simulink model "psbloadshed"  (Simulink 6.0)
settings: Solver=ode23tb  SolverMode=SingleTasking  StartTime=0.0  StopTime=2  RelTol=1e-3
InitFcn:
  | powericon('psbinitsys',bdroot);
libraries: powerlib2 x9, simulink x1
settings Model: Creator=patrice  LastModifiedBy=batserve  ExtModeTrigMode=oneshot  ExtModeArmWhenConnect=off  ExtModeAutoUpdateStatusClock=off
settings DataIOCC: LimitDataPoints=off  SignalLoggingName=sigsOut
settings OptimizationCC: BlockReduction=off  BooleanDataType=off
settings DebuggingCC: CheckExecutionContextPreStartOutputMsg=on  CheckExecutionContextRuntimeOutputMsg=on  SolverPrmCheckMsg=none  IntegerOverflowMsg=none
settings HardwareCC: TargetUnknown=on
settings RTWCC: TemplateMakefile=grt_unix.tmf

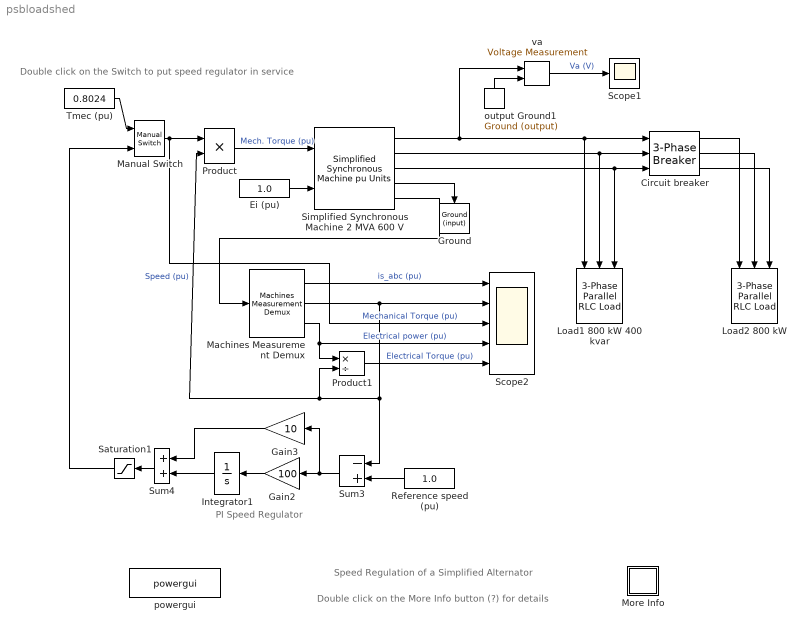
== system psbloadshed ==
  note: Speed Regulation of a Simplified Alternator
  note: Double click on the More Info button (?) for details
  note: PI Speed Regulator
  note: Double click on the  Switch
      | to put speed regulator
      | in service
  Circuit breaker : powerlib2/Elements/3-Phase Breaker  init_states=closed  sa=on  sb=on  sc=on  sw_times=[ 0.2 0.7*100 ]  Ts=0  comext=off  Ron=1e-4  Rp=inf  Cp=0  mesure=None
  Ei (pu) : Constant  Value=1.0
  Gain2 : Gain  Orientation=left  Gain=100  SaturateOnIntegerOverflow=on
  Gain3 : Gain  Orientation=left  Gain=10  SaturateOnIntegerOverflow=on
  Ground : powerlib2/Connectors/Ground (input)  Tag=PoWeRsYsTeMbLoCk  Orientation=down
  Integrator1 : Integrator  Orientation=left  InitialCondition=0.8024  LimitOutput=on  UpperSaturationLimit=1  LowerSaturationLimit=0  ZeroCross=off
  Load1 800 kW 400 kvar : powerlib2/Elements/3-Phase Parallel RLC Load  Orientation=down  Vpp=600  fn=60  P3=800e3  QL3=400e3  QC3=0
  Load2 800 kW : powerlib2/Elements/3-Phase Parallel RLC Load  Orientation=down  Vpp=600  fn=60  P3=800e3  QL3=0  QC3=0
  Machines Measurement Demux : powerlib2/Machines/Machines Measurement Demux  machType=Simplified synchronous  ssm1=on  ssm2=off  ssm3=off  ssm4=off  ssm5=on  ssm6=on  sm1=on  sm2=on  sm3=on  sm4=on  sm5=on  sm6=on  sm7=on  sm8=on  sm9=on  sm10=on  sm11=on  sm115=off  sm12=off  sm13=off  sm14=off  asm1=on  asm2=on  asm3=on  asm4=on  asm5=on  asm6=on  asm7=on  asm8=on  asm9=on  asm10=on  asm11=on  pmsm1=on  pmsm2=on  pmsm3=on  pmsm4=on  pmsm5=on  pmsm6=on  lastType=1
  Manual Switch : simulink/Signal Routing/Manual Switch  sw=1  action=0
  More Info : Subsystem
      mask Display: disp('?')
  Product : Product  SaturateOnIntegerOverflow=on  InputSameDT=on
  Product1 : Product  Inputs=*/  SaturateOnIntegerOverflow=on  InputSameDT=on
  Reference speed (pu) : Constant  Orientation=left  Value=1.0
  Saturation1 : Saturate  Orientation=left  UpperLimit=1  LowerLimit=0  ZeroCross=off
  "Scope1 " : Scope
      settings: TimeRange=0.2  YMin=-500  YMax=500  DataFormat=Structure
  Scope2 : Scope  NumInputPorts=5
      settings: TimeRange=2  YMin=-1~1~-2~0~0  YMax=1~2~2~1~1  DataFormat=Structure  SampleTime=1/60
  Simplified Synchronous Machine 2 MVA 600 V : powerlib2/Machines/Simplified Synchronous  Machine  pu Units  Tag=PoWeRsYsTeMbLoCk  conType=4-wire Y  x1="[  2000e3, 600, 60 ]"  x2=[ 0.6 , 0.0, 2 ]  x3="[ 0.0036  0.16 ]"  x4="[0 0  0 0 0    0  0  0]"  PSBOutputType=11110  iounits=0  LoadFlowParameters=[2 0 0 0]
  Sum3 : Sum  Orientation=left  Inputs=-+  SaturateOnIntegerOverflow=on  InputSameDT=on
  Sum4 : Sum  Orientation=left  SaturateOnIntegerOverflow=on  InputSameDT=on
  Tmec (pu) : Constant  Value=0.8024
  output Ground1 : powerlib2/Connectors/Ground (output)  Tag=PoWeRsYsTeMbLoCk  Orientation=up  PSBOutputType=1
  powergui : powerlib2/powergui  Frange=[0:2:500]  Ylog=off  Xlog=on  save=off  variable=ZData  ZoomFFT=on  StartTime=0.0  cycles=1  DisplayStyle=off  fundamental=60  FreqAxis=off  MaxFrequency=1000  frequencyindice=1  frequencyindicesteady=1  RmsSteady=1  display=off  Ts=0  methode=off  frequency=60  echomessages=off
  va : powerlib2/Measurements/Voltage Measurement  Tag=PoWeRsYsTeMmEaSuReMeNt  PhasorSimulation=off  OutputType=Magnitude  PSBOutputType=0  PSBequivalent=0
  wires:
  Simplified Synchronous Machine 2 MVA 600 V/5 -> Machines Measurement Demux/1
  Circuit breaker/1 -> Load2 800 kW/1
  Ei (pu)/1 -> Simplified Synchronous Machine 2 MVA 600 V/2
  Circuit breaker/2 -> Load2 800 kW/2
  Circuit breaker/3 -> Load2 800 kW/3
  Simplified Synchronous Machine 2 MVA 600 V/2 -> Circuit breaker/2, Load1 800 kW 400 kvar/2
  Simplified Synchronous Machine 2 MVA 600 V/3 -> Load1 800 kW 400 kvar/3, Circuit breaker/3
  Simplified Synchronous Machine 2 MVA 600 V/1 -> Circuit breaker/1, Load1 800 kW 400 kvar/1, va/1
  output Ground1/1 -> va/2
  Machines Measurement Demux/1 -> Scope2/1  "is_abc (pu)"
  Machines Measurement Demux/2 -> Scope2/2, Sum3/1, Product/2, Product1/2  "Speed (pu)"
  Gain3/1 -> Sum4/1
  Gain2/1 -> Integrator1/1
  Sum3/1 -> Gain3/1, Gain2/1
  Integrator1/1 -> Sum4/2
  Reference speed (pu)/1 -> Sum3/2
  Sum4/1 -> Saturation1/1
  Product/1 -> Simplified Synchronous Machine 2 MVA 600 V/1  "Mech. Torque (pu)"
  va/1 -> "Scope1 "/1  "Va (V)"
  Tmec (pu)/1 -> Manual Switch/1
  Manual Switch/1 -> Product/1, Scope2/3  "Mechanical Torque (pu)"
  Saturation1/1 -> Manual Switch/2
  Machines Measurement Demux/3 -> Product1/1, Scope2/4  "Electrical power (pu)"
  Product1/1 -> Scope2/5  "Electrical Torque (pu)"
  Simplified Synchronous Machine 2 MVA 600 V/4 -> Ground/1

== system psbloadshed/More Info ==
  note: 2. Simulation at constant torque - No speed regulator
  note: 1. Initializing the machine to start in steady state
  note: Demonstration
  note: Circuit Description
  note: This demonstration illustrates the  use of the simplified alternator
      | for a load shedding test on a 2000 kVA, 600 V alternator.
  note: Make sure that the speed regulator is not in service ( Manual Switch is in the upper position) . Start the simulation and observe signals on Scope2.
      | The three Iabc currents should start with steady-state sinusoidal waveforms.  Observe that when the circuit breaker  opens  at t = 0.2 s, the electrical power (trace 4)
      | drops from 0.8 pu to 0.4 pu and  that the machine starts to accelerate.The rate of speed increase is dN/dt = 1/2H = 0.833 pu speed/ pu torque / s.
      | As the net electromechanical torque is now Tmec-Telec = 0.8 - 0.4 = 0.4 pu, the speed increases at a rate of 0.833*0.4 = 0.33 pu/s.  At t = 1.2s, the expected speed increase
      | is therefore 0.33 pu. In fact, the  speed measured  at t = 1.2 s is slightly higher than the theoretical value (1.38 pu as compared to 1.33 pu).
      | This is because the electrical torque (trace 5) decreases as speed is increasing, resulting in a net acceleration torque higher than 0.4 pu.
  note: A three-phase, four-wire alternator rated 2000 kVA, 1600 kW, 0.8 power factor, 600 V, 1800 rpm  is connected to a 1600 kW, 400 kvar inductive load.
      | The stator neutral point is grounded. The internal impedance of the generator (Zg = 0.0036 + j*0.16 pu) represents the armature winding
      | resistance Ra and direct axis transient reactance X'd. The total inertia constant  of the generator and prime mover  is H = 0.6 s, corresponding to J = 67.5 kg.m^2.
      | Speed regulation is modelled with  Simulink blocks implementing a PI regulator. The machine is excited with a constant voltage.
      |
      | A three-phase breaker is used to switch out a 800 kW resistive load. The breaker is initially closed and it is opened at t = 0.2 s, resulting in  a 50% load shedding.
      | In this demo you will learn how to initialize the machine in order start simulation in steady state and you will observe the machine dynamics with and without speed regulation.
  note: Start Simulation and observe the three machine currents on trace 1 of Scope2. If  the 8 parameters defining initial conditions  for the machine are left at zero or not set
      | correctly , the simulation will not start in steady state. In order to start the simulation in steady-state you must first initialize the machine for the desired load flow.
      |
      | Open the powergui and select 'Load Flow & Machine Initialization'.  A new  window appears. As your circuit contains no voltage source
      | imposing the reference angle, you must select  'Swing Bus'  for the machine 'Bus type'.  This means that  the load flow will be performed with the machine
      | controlling the voltage and the angle at its terminals. The desired terminal  voltage  should be already initialized at 600 V (machine nominal voltage); leave
      | the phase angle of UAN angle at 0 degree and do not specify any power guess. Then press the 'Execute Load Flow' button.
      |
      | Once the load flow is solved the three line-to-line machine voltages as well as the three machine output  currents   are updated.
      | The machine active and  reactive powers as well as  the required  mechanical power Pmec and  field voltage E  are also displayed.
      | You should get the following values : P = 1600kW, Q = 400 kvar, Pmec = 1604.7kW (0.8024 pu),  field voltage E = 1.0247 pu. The Load Flow also prompts
      | you with a warning to set initial condition for mechanical power to 0.8024 pu. This is because the Pm input of the machine  is not connected to a
      | constant block or to a library block  (HTG or STG ). Notice that the mechanical torque (Tmec block) is already set at 0.8024 pu. Disregard this message.
      | Notice  also that the constant block Ei connected at the E input of the machine is automatically updated (E = 1.04268 pu).
  note: G. Sybille (Hydro-Quebec)
  note: 3. Simulation with speed regulator
  note: Now double click on the Manual Switch block  in order to put the speed regulator in service. Restart the simulation and observe the dynamic response of the speed
      | regulator on Scope 2. Notice that in order to maintain speed at its reference value (1 pu), the speed regulator has reduced the mechanical torque to 0.4 pu.
